simulink model "early_late"  (Simulink 6.6)
settings: Solver=VariableStepDiscrete  StartTime=0.0  StopTime=5000  RelTol=1e-3
PreLoadFcn:
  | Fs = 1;
StopFcn:
  | figure(1)
  | plot(ted_output);
  | legend('Timing Error Detector Output',1);
  | xlabel('Samples');
  | ylabel('Amplitude');
  | 
  | figure(2)
  | hold off
  | plot(Vss_nom,'b');
  | hold on
  | plot(Vss,'r');
  | legend('Nominal SS', 'Adj. SS',0);
  | xlabel('Samples');
  | ylabel('Step Size');
  | 
  | figure(3)
  | hold off
  | plot(mf_signal,'k-');
  | hold on
  | plot(sample_points,'r-o');
  | plot(zeros(1,length(mf_signal)),'k--');
  | legend('Input','Samples',4)
  | axis([0 length(mf_signal) 1.2*min(mf_signal) 1.2*max(mf_signal)]);
  | xlabel('Samples');
  | ylabel('Amplitude');
undefined symbols (not defined in the file): dfilt
libraries: xbsIndex_r4 x27, dspsrcs4 x1, dsparch4 x1, dspsigops x1
settings Model: Creator=lcrockett  LastModifiedBy=lcrockett

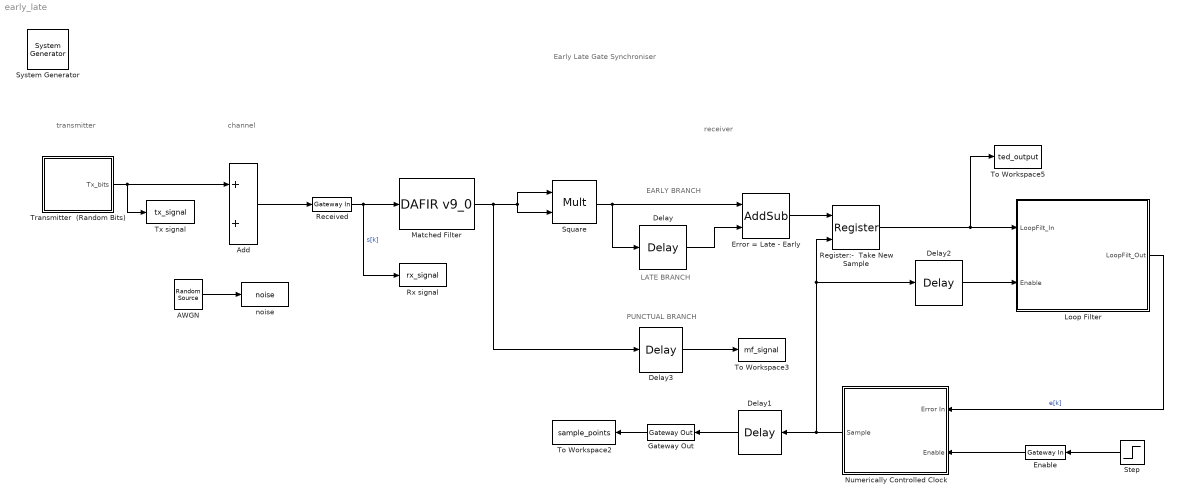
== system early_late ==
  note: Early Late Gate Synchroniser
  note: transmitter
  note: channel
  note: LATE BRANCH
  note: EARLY BRANCH
  note: receiver
  note: PUNCTUAL BRANCH
  " System Generator" : xbsIndex_r4/ System Generator  Tag=genX  SystemSampleTime=-1  xilinxfamily=virtex4  part=xc4vsx35  speed=-10  package=ff668  synthesis_tool=XST  clock_wrapper=Clock Enables  directory=./netlist  testbench=off  simulink_period=1/Fs  sysclk_period=10  dcm_input_clock_period=100  incr_netlist=off  trim_vbits=Everywhere in SubSystem  dbl_ovrd=According to Block Masks  core_generation=According to Block Masks  run_coregen=off  deprecated_control=off  eval_field=0  block_type=sysgen
      settings: block_version=9.2.01
  AWGN : dspsrcs4/Random Source  SrcType=Gaussian  NormMethod=Ziggurat  CltLength=12  MinVal=0  MaxVal=1  MeanVal=0  VarVal=0.2  RepMode=Not repeatable  rawSeed=1  IsInherit=on  SampMode=Discrete  SampTime=1  SampFrame=1  DataType=Single  OutComplex=Real
  Add : Sum  OutDataTypeMode=double  OutScaling=2^-10
  Delay : xbsIndex_r4/Delay  en=off  latency=10  dbl_ovrd=off  reg_retiming=off  block_type=delay
      settings: block_version=9.2.01
  Delay1 : xbsIndex_r4/Delay  Orientation=left  en=off  latency=10  dbl_ovrd=off  reg_retiming=off  block_type=delay
      settings: block_version=9.2.01
  Delay2 : xbsIndex_r4/Delay  en=off  latency=1  dbl_ovrd=off  reg_retiming=off  block_type=delay
      settings: block_version=9.2.01
  Delay3 : xbsIndex_r4/Delay  en=off  latency=5  dbl_ovrd=off  reg_retiming=off  block_type=delay
      settings: block_version=9.2.01
  Enable : xbsIndex_r4/Gateway In  Orientation=left  arith_type=Boolean  n_bits=16  bin_pt=14  quantization="Round  (unbiased: +/- Inf)"  overflow=Saturate  period=1/Fs  dbl_ovrd=off  timing_constraint=None  locs_specified=off  LOCs={}  block_type=gatewayin
      settings: infoedit="Gateway in block.  Converts inputs of type Simulink integer, double and fixed point to  Xilinx fixed point type.<P><P>Hardware notes:  In hardware these blocks become top level input ports."  block_version=9.2.01
  Error = Late - Early : xbsIndex_r4/AddSub  mode=Subtraction  use_carryin=off  use_carryout=off  en=off  latency=0  precision=Full  arith_type=Unsigned  n_bits=16  bin_pt=14  quantization=Truncate  overflow=Wrap  dbl_ovrd=off  use_behavioral_HDL=off  pipelined=off  use_rpm=on  block_type=addsub
      settings: block_version=9.2.01
  Gateway Out : xbsIndex_r4/Gateway Out  Orientation=left  hdl_port=on  timing_constraint=None  locs_specified=off  LOCs={}  block_type=gatewayout
      settings: infoedit="Gateway out block.  Converts Xilinx fixed point inputs into ouputs of type Simulink integer, double, or fixed point.<P><P>Hardware notes:  In hardware these blocks become top level output ports or are discarded, depending on how they are configured."  block_version=9.2.01
  Loop Filter : Subsystem  mask(Loop Filter Parameters){alpha_n=3, beta_n=7, phase_det_word=16, extend_wl=on}
      mask prompts: alpha_n "Alpha (bits to shift right by)"; beta_n "Beta (bits to shift right by)"; phase_det_word "Input wordlength"; extend_wl "Retain full precision?"
      mask help:
      | The loop filter contains two paths: a proportional path and an integral path. These are characterised by coefficients Alpha and Beta, respectively. Multiplications by these coefficients are both realised via shifts, for hardware efficiency reasons.
      |
      | Mask to be completed... not yet straight on the wordlength implications and the choices that should be presented via the mask.
      mask init:
      | if extend_wl == true
      |     alpha_shift_wl = phase_det_word + alpha_n;
      |     beta_shift_wl = phase_det_word + beta_n;
      | else
      |     alpha_shift_wl = phase_det_word;
      |     beta_shift_wl = phase_det_word;
      | end
  "Matched Filter " : xbsIndex_r4/DAFIR v9_0   coef=(1/20)*ones(1,20)  structure=Inferred from Coefficients  coef_n_bits=16  coef_bin_pt=14  over_sample=1  reload=off  valids=off  rst=off  latency=1  num_channels=1  serial_input=off  polyphase_behavior="Single Rate:  sample in - sample out"  dbl_ovrd=off  explicit_period=off  period=1  use_isim=0  block_type=fir
      settings: infoedit="Hardware notes: Implemented using distributed arithmetic (DA).  The hardware over sampling rate determines the degree of parallelism.  A rate of one produces a fully parallel DA filter.  A rate of n (resp., n+1) for an n-bit input signal produces a fully serial implementation for a non-symmetric (resp., symmetric) impulse response.  Intermediate values produce implementations with intermediate levels of parallelism."  block_version=9.2.01
  Numerically Controlled Clock : Subsystem  Orientation=left  mask(Numerically Controlled Clock (NCC)){N=256, F_res=0.000001, F_nom=1/20, F_s=Fs}
      mask prompts: N "Counter Size"; F_res "Desired Frequency Resolution (Hz)"; F_nom "Nominal Rate/Frequency"; F_s "Sampling Frequency (Hz)"
      mask help: This component operates similarly to an NCO. Its "centre" rate is supplied by the user, defining the nominal step size applied to an accumulator. In operation, the control input "Error In" supplies a step size adjustment, which is applied to the nominal step size and input to an accumulator. When the accumulator wraps, a sample is taken (i.e. a single cycle 1 output).
      mask init:
      | delta_mu_des = (F_res * N) / F_s;
      | fract_bits = ceil(abs((log10(delta_mu_des) / log10(2))));
      | whole_bits = round(log(N)/log(2));
      | mu_nom = (F_nom * N) / F_s;
      | F_res_act = F_s / ((2^fract_bits) * N);
  Received : xbsIndex_r4/Gateway In  arith_type="Signed  (2's comp)"  n_bits=20  bin_pt=14  quantization="Round  (unbiased: +/- Inf)"  overflow=Saturate  period=1/Fs  dbl_ovrd=off  timing_constraint=None  locs_specified=off  LOCs={}  block_type=gatewayin
      settings: infoedit="Gateway in block.  Converts inputs of type Simulink integer, double and fixed point to  Xilinx fixed point type.<P><P>Hardware notes:  In hardware these blocks become top level input ports."  block_version=9.2.01
  Register:-  Take New Sample : xbsIndex_r4/Register  init=0  rst=off  en=on  dbl_ovrd=off  block_type=register
      settings: block_version=9.2.01
  Rx signal : ToWorkspace  VariableName=rx_signal  SampleTime=1  SaveFormat=Array
  Square : xbsIndex_r4/Mult  precision=Full  arith_type="Signed  (2's comp)"  n_bits=16  bin_pt=14  quantization=Truncate  overflow=Wrap  en=off  latency=0  dbl_ovrd=off  use_behavioral_HDL=off  use_embedded=on  opt=Speed  optimum_pipeline=off  pipeline=on  use_rpm=on  placement_style=Triangular  block_type=mult
      settings: infoedit=Hardware notes: To use the internal pipeline stage of the dedicated multiplier you must select 'Pipeline for maximum performance'.  block_version=9.2.01
  Step : Step  Orientation=left  Time=3  SampleTime=Fs
  To Workspace2 : ToWorkspace  VariableName=sample_points  SampleTime=-1  SaveFormat=Array
  To Workspace3 : ToWorkspace  VariableName=mf_signal  SampleTime=-1  SaveFormat=Array
  To Workspace5 : ToWorkspace  VariableName=ted_output  SampleTime=-1  SaveFormat=Array
  Transmitter  (Random Bits) : Subsystem  mask(Random Source){s=20}
      mask prompts: s "Samples per bit (integer)"
      mask help: This random source has rectangular pulse shaping, and the length of each bit can be specified in samples (this must be an integer).
  Tx signal : ToWorkspace  VariableName=tx_signal  SampleTime=1  SaveFormat=Array
  noise : ToWorkspace  VariableName=noise  SampleTime=1  SaveFormat=Array
  wires:
  Loop Filter/1(LoopFilt_Out) -> Numerically Controlled Clock/1(Error In)  "e[k]"
  Received/1 -> "Matched Filter "/1, Rx signal/1  "s[k]"
  Gateway Out/1 -> To Workspace2/1
  Register:-  Take New Sample/1 -> Loop Filter/1(LoopFilt_In), To Workspace5/1
  Add/1 -> Received/1
  Transmitter  (Random Bits)/1(Tx_bits) -> Add/1, Tx signal/1
  AWGN/1 -> noise/1
  Delay/1 -> Error = Late - Early/2
  Error = Late - Early/1 -> Register:-  Take New Sample/1
  "Matched Filter "/1 -> Square/1, Square/2, Delay3/1
  Square/1 -> Error = Late - Early/1, Delay/1
  Numerically Controlled Clock/1(Sample) -> Delay1/1, Register:-  Take New Sample/2, Delay2/1
  Enable/1 -> Numerically Controlled Clock/2(Enable)
  Step/1 -> Enable/1
  Delay1/1 -> Gateway Out/1
  Delay2/1 -> Loop Filter/2(Enable)
  Delay3/1 -> To Workspace3/1

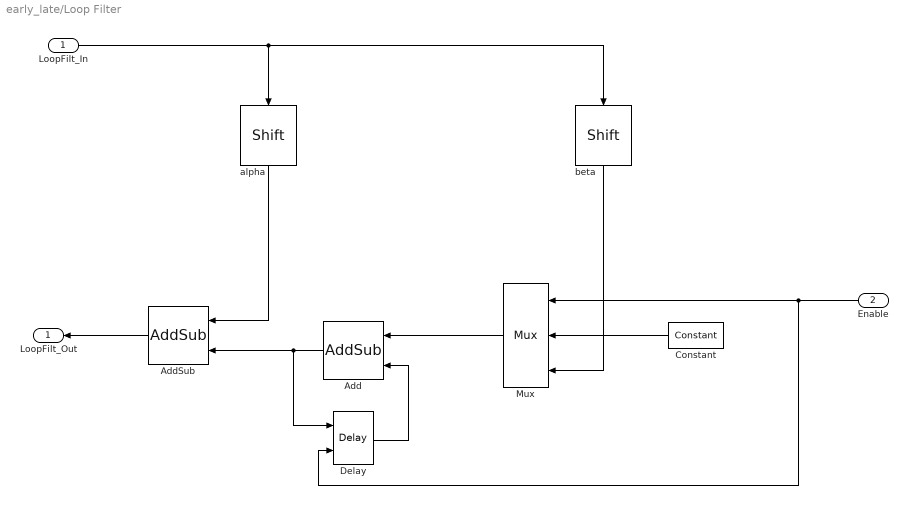
== system early_late/Loop Filter ==
  LoopFilt_In : Inport
  Enable : Inport  Orientation=left  Port=2
  Add : xbsIndex_r4/AddSub  Orientation=left  mode=Addition  use_carryin=off  use_carryout=off  en=off  latency=0  precision=User Defined  arith_type="Signed  (2's comp)"  n_bits=40  bin_pt=20  quantization="Round  (unbiased: +/- Inf)"  overflow=Wrap  dbl_ovrd=off  use_behavioral_HDL=off  pipelined=off  use_rpm=on  block_type=addsub
      settings: block_version=9.2.01
  AddSub : xbsIndex_r4/AddSub  Orientation=left  mode=Addition  use_carryin=off  use_carryout=off  en=off  latency=0  precision=Full  arith_type="Signed  (2's comp)"  n_bits=20  bin_pt=14  quantization="Round  (unbiased: +/- Inf)"  overflow=Wrap  dbl_ovrd=off  use_behavioral_HDL=off  pipelined=off  use_rpm=on  block_type=addsub
      settings: block_version=9.2.01
  Constant : xbsIndex_r4/Constant  Orientation=left  arith_type=Signed (2's comp)  const=0  n_bits=2  bin_pt=0  explicit_period=off  period=1  equ=P=C  opselect=C  inp2=PCIN>>17  opr=+  inp1=P  carry=CIN  dbl_ovrd=off  block_type=constant
      settings: block_version=9.2.01
  Delay : xbsIndex_r4/Delay  en=on  latency=1  dbl_ovrd=off  reg_retiming=off  block_type=delay
      settings: block_version=9.2.01
  Mux : xbsIndex_r4/Mux  Orientation=left  inputs=2  en=off  latency=0  precision=Full  arith_type=Unsigned  n_bits=16  bin_pt=14  quantization=Truncate  overflow=Wrap  dbl_ovrd=off  block_type=mux
      settings: block_version=9.2.01
  alpha : xbsIndex_r4/Shift  Orientation=down  shift_dir=Right  shift_bits=alpha_n  en=off  latency=0  precision=User Defined  arith_type="Signed  (2's comp)"  n_bits=alpha_shift_wl  bin_pt=alpha_shift_wl-2  quantization="Round  (unbiased: +/- Inf)"  overflow=Wrap  dbl_ovrd=off  block_type=shift
      settings: block_version=9.2.01
  beta : xbsIndex_r4/Shift  Orientation=down  shift_dir=Right  shift_bits=beta_n  en=off  latency=0  precision=User Defined  arith_type="Signed  (2's comp)"  n_bits=beta_shift_wl  bin_pt=beta_shift_wl-2  quantization="Round  (unbiased: +/- Inf)"  overflow=Wrap  dbl_ovrd=off  block_type=shift
      settings: block_version=9.2.01
  LoopFilt_Out : Outport  Orientation=left
  wires:
  Add/1 -> AddSub/2, Delay/1
  alpha/1 -> AddSub/1
  Delay/1 -> Add/2
  LoopFilt_In/1 -> alpha/1, beta/1
  AddSub/1 -> LoopFilt_Out/1
  beta/1 -> Mux/3
  Mux/1 -> Add/1
  Enable/1 -> Mux/1, Delay/2
  Constant/1 -> Mux/2

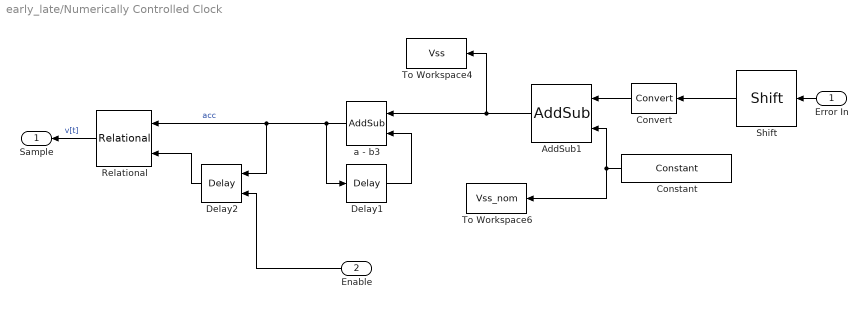
== system early_late/Numerically Controlled Clock ==
  Error In : Inport  Orientation=left
  Enable : Inport  Orientation=left  Port=2
  AddSub1 : xbsIndex_r4/AddSub  Orientation=left  mode=Addition  use_carryin=off  use_carryout=off  en=off  latency=0  precision=User Defined  arith_type=Unsigned  n_bits=whole_bits + fract_bits  bin_pt=fract_bits  quantization="Round  (unbiased: +/- Inf)"  overflow=Wrap  dbl_ovrd=off  use_behavioral_HDL=off  pipelined=off  use_rpm=on  block_type=addsub
      settings: block_version=9.2.01
  Constant : xbsIndex_r4/Constant  Orientation=left  arith_type=Unsigned  const=mu_nom  n_bits=whole_bits + fract_bits  bin_pt=fract_bits  explicit_period=on  period=1/Fs  equ=P=C  opselect=C  inp2=PCIN>>17  opr=+  inp1=P  carry=CIN  dbl_ovrd=off  block_type=constant
      settings: block_version=9.2.01
  Convert : xbsIndex_r4/Convert  Orientation=left  arith_type="Signed  (2's comp)"  n_bits=whole_bits+fract_bits  bin_pt=fract_bits  quantization=Truncate  overflow=Wrap  latency=0  dbl_ovrd=off  pipeline=off  block_type=convert
      settings: block_version=9.2.01
  Delay1 : xbsIndex_r4/Delay  en=off  latency=1  dbl_ovrd=off  reg_retiming=off  block_type=delay
      settings: block_version=9.2.01
  Delay2 : xbsIndex_r4/Delay  Orientation=left  en=on  latency=1  dbl_ovrd=off  reg_retiming=off  block_type=delay
      settings: block_version=9.2.01
  Relational : xbsIndex_r4/Relational  Orientation=left  mode=a<b  en=off  latency=1  dbl_ovrd=off  block_type=relational
      settings: block_version=9.2.01
  Shift : xbsIndex_r4/Shift  Orientation=left  shift_dir=Left  shift_bits=4  en=off  latency=0  precision=Full  arith_type="Signed  (2's comp)"  n_bits=16  bin_pt=14  quantization=Truncate  overflow=Wrap  dbl_ovrd=off  block_type=shift
      settings: block_version=9.2.01
  To Workspace4 : ToWorkspace  VariableName=Vss  SampleTime=-1  SaveFormat=Array
  To Workspace6 : ToWorkspace  VariableName=Vss_nom  SampleTime=-1  SaveFormat=Array
  a - b3 : xbsIndex_r4/AddSub  Orientation=left  mode=Addition  use_carryin=off  use_carryout=off  en=off  latency=0  precision=User Defined  arith_type=Unsigned  n_bits=whole_bits + fract_bits  bin_pt=fract_bits  quantization=Truncate  overflow=Wrap  dbl_ovrd=off  use_behavioral_HDL=off  pipelined=off  use_rpm=on  block_type=addsub
      settings: block_version=9.2.01
  Sample : Outport  Orientation=left
  wires:
  a - b3/1 -> Delay1/1, Delay2/1, Relational/1  "acc"
  Delay1/1 -> a - b3/2
  AddSub1/1 -> a - b3/1, To Workspace4/1
  Constant/1 -> AddSub1/2, To Workspace6/1
  Delay2/1 -> Relational/2
  Error In/1 -> Shift/1
  Relational/1 -> Sample/1  "v[t]"
  Enable/1 -> Delay2/2
  Convert/1 -> AddSub1/1
  Shift/1 -> Convert/1

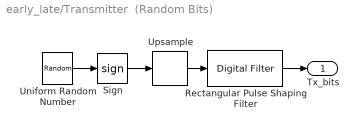
== system early_late/Transmitter  (Random Bits) ==
  Rectangular Pulse Shaping Filter : dsparch4/Digital Filter  DialogController=dspdialog.DigitalFilter  DialogControllerArgs=DataTag2  TypePopup=FIR (all zeros)  IIRFiltStruct=Direct form II transposed  AllPoleFiltStruct=Direct form  FIRFiltStruct=Direct form  CoeffSource=Specify via dialog  NumCoeffs=ones(1,s)  DenCoeffs=[1 0.1]  BiQuadCoeffs=[1 0.3 0.4 1 0.1 0.2]  LatticeCoeffs=[0.2 0.4]  denIgnore=on  FiltPerSampPopup=One filter per frame  IC=0  ICnum=0  ICden=0  roundingMode=Floor  overflowMode=off  ScaleValues=1  scaleValueFracLength=14  stageInFracLength=15  stageOutFracLength=15  FilterSource=Specify via dialog  dfiltObjectName=dfilt.dffir([1 2 1])
  Sign : Signum
  Uniform Random Number : UniformRandomNumber  Seed=546  SampleTime=s
  Upsample : dspsigops/Upsample  N=s  phase=0  ic=0  mode=Maintain input frame size
  Tx_bits : Outport
  wires:
  Uniform Random Number/1 -> Sign/1
  Sign/1 -> Upsample/1
  Upsample/1 -> Rectangular Pulse Shaping Filter/1
  Rectangular Pulse Shaping Filter/1 -> Tx_bits/1
